simulink model "Copy_of_dwa_r2015a"  (R2015a)
settings: Solver=ode45  StartTime=0.0  StopTime=10.0  RelTol=1e-3
values from neighbouring files (symbols this model uses):
  c = 3.5e-2    (= 0.035)    [main.m]
  k = 42    [main.m]    (also in test_usw.m = [3,0.1])
  k_ac = 51    [main.m]
  k_af = 2.59e-2    (= 0.0259)    [main.m]
  m_c = 8.5    [main.m]
  m_f = 0.7e-3    (= 0.0007)    [main.m]
undefined symbols (not defined in the file or in its folder): sigbuilder_block
settings Model: CovModelRefEnable=off  Creator=chao  LastModifiedBy=chao
settings DataIOCC: LimitDataPoints=off  SaveFormat=Dataset
settings HardwareCC: ProdBitPerPointer=64  ProdLargestAtomicFloat=Float  ProdIntDivRoundTo=Zero  ProdEndianess=LittleEndian  ProdHWDeviceType=Specified
settings ModelReferenceCC: PropagateSignalLabelsOutOfModel=on
settings GRTTargetCC: GeneratePreprocessorConditionals=Use local settings

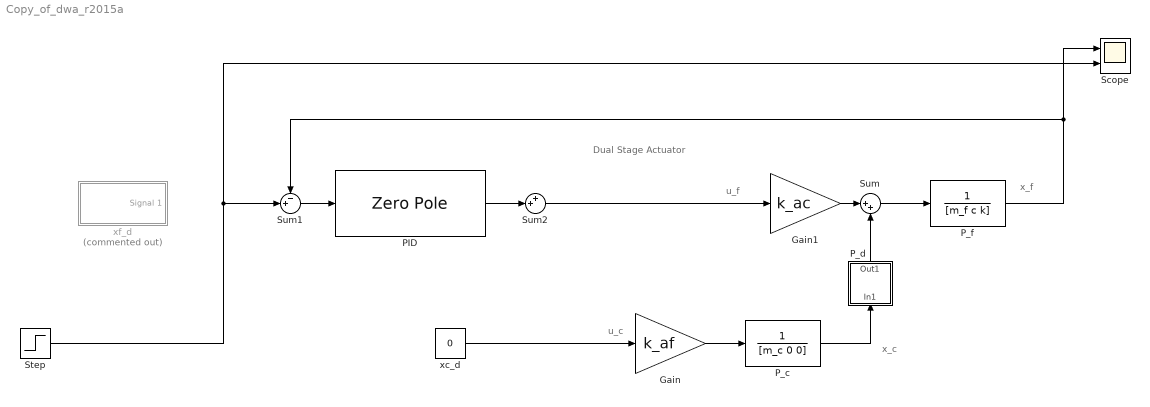
== system Copy_of_dwa_r2015a ==
  note: Dual Stage Actuator
  note: u_f
  note: u_c
  note: x_c
  note: x_f
  Gain : Gain  Gain=k_af
  Gain1 : Gain  Gain=k_ac
  PID : ZeroPole  Zeros=[-2*pi*100 -2*pi*333]  Poles=[0 -2*pi*3000]  Gain=[3.2e6]
  P_c : TransferFcn  Denominator=[m_c 0 0]
  P_d : Subsystem
  P_f : TransferFcn  Denominator=[m_f c k]
  Scope : Scope  NumInputPorts=2
      settings: TimeRange=auto  MaxDataPoints=5000  SaveToWorkspace=off  SaveName=ScopeData  YMin=-0.00024~-5  YMax=0.00217~5  SampleTime=-1
  Step : Step  After=1e-3  SampleTime=0
  Sum : Sum  Inputs=|++
  Sum1 : Sum  Inputs=-+|
  Sum2 : Sum  Inputs=++|
  xc_d : Constant  Value=0
  xf_d : Subsystem  Tag=STV Subsys  Commented=on  LoadFcn=sigbuilder_block('load');  StartFcn=sigbuilder_block('start');  StopFcn=sigbuilder_block('stop');  ClipboardFcn=sigbuilder_block('clipboard');  mask(Sigbuilder block){}
      mask help: Simulink:masks:SigbuilderBlock_MD
      mask init:
      | if ~strcmp(get_param(bdroot(gcbh),'SimulationStatus'),'stopped') tuvar = sigbuilder_block('maskInit'); end
      settings: CopyFcn=sigbuilder_block('copy');  DeleteFcn=sigbuilder_block('delete');  ModelCloseFcn=sigbuilder_block('modelClose');  PreSaveFcn=sigbuilder_block('preSave');  PauseFcn=sigbuilder_block('pause');  ContinueFcn=sigbuilder_block('continue');  NameChangeFcn=sigbuilder_block('namechange');  OpenFcn=sigbuilder_block('open',[437.4 192 550.8 400.2 ]);  CloseFcn=sigbuilder_block('close');
      mask Display: plot(0, 0, 100, 100,[2, 2, 32, 32, 2], [68, 8, 8, 68, 68],[32, 2], [38, 38], [32, 19, 2],[53, 60, 44], [32, 17, 17, 2],[16, 16, 31, 31]);txt = getActiveGroup(gcbh);text(2, 100, txt,'verticalAlignment', 'top');
  wires:
  Gain1/1 -> Sum/1
  Sum/1 -> P_f/1
  P_d/1(Out1) -> Sum/2
  P_c/1 -> P_d/1(In1)
  Gain/1 -> P_c/1
  Sum1/1 -> PID/1
  PID/1 -> Sum2/2
  Sum2/1 -> Gain1/1
  xc_d/1 -> Gain/1
  P_f/1 -> Scope/1, Sum1/1
  Step/1 -> Scope/2, Sum1/2

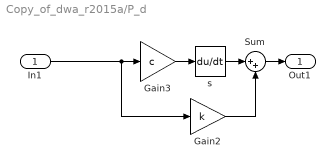
== system Copy_of_dwa_r2015a/P_d ==
  In1 : Inport
  Gain2 : Gain  Gain=k
  Gain3 : Gain  Gain=c
  Sum : Sum  Inputs=|++
  s : Derivative
  Out1 : Outport
  wires:
  Sum/1 -> Out1/1
  Gain2/1 -> Sum/2
  s/1 -> Sum/1
  Gain3/1 -> s/1
  In1/1 -> Gain2/1, Gain3/1

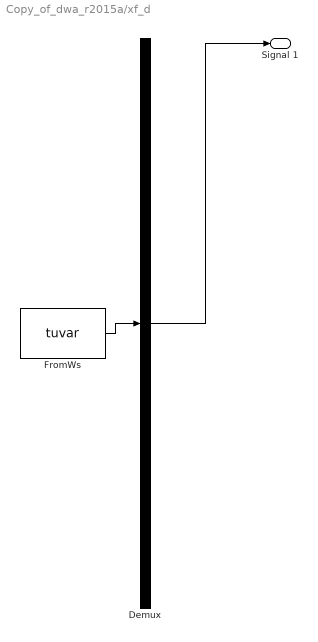
== system Copy_of_dwa_r2015a/xf_d ==
  Demux : Demux  Tag=STV Demux  Outputs=1
  FromWs : FromWorkspace  Tag=STV FromWs  VariableName=tuvar  SampleTime=0
      SigBuilderData=|
      | common.afterFinalStr = 'Extrapolate'
      | common.sampleTime = 0
      | dataSet.timeRange = [0 10]
      | dataSet.name = 'Group 1'
      | sbobj.Groups.Name = 'Group 1'
      | sbobj.Groups.Signals.Name = 'Signal 1'
      | sbobj.Groups.Signals.XData = [0 1 4 5 8 10]
      | sbobj.Groups.Signals.YData = [0 0 0.001 0.001 0 0]
  Signal 1 : Outport  Tag=STV Outport
  wires:
  Demux/1 -> Signal 1/1
  FromWs/1 -> Demux/1
